simulink model "astatismo"  (R2026a)
settings: Solver=VariableStepAuto  StopTime=12  MaxStep=1e-2  RelTol=1e-6
undefined symbols (not defined in the file): A, B, C, C_theta, C_x, K_aum_2
settings Model: Creator=matte  LastModifiedBy=matte
settings OptimizationCC: BooleanDataType=off
settings DebuggingCC: SaveWithParameterizedLinksMsg=none  SignalResolutionControl=TryResolveAllWithWarning
settings HardwareCC: TargetUnknown=on

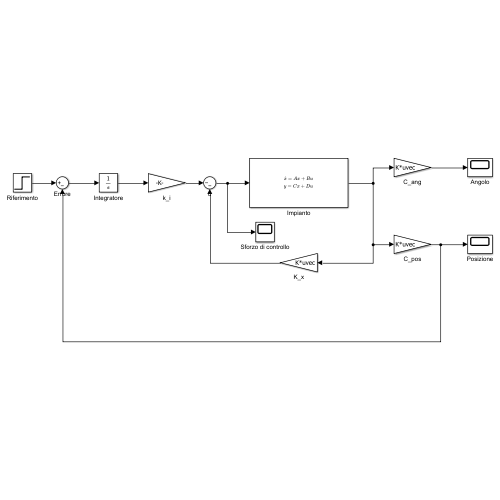
[thumbnail: Simulink's stored preview of the top-level diagram]
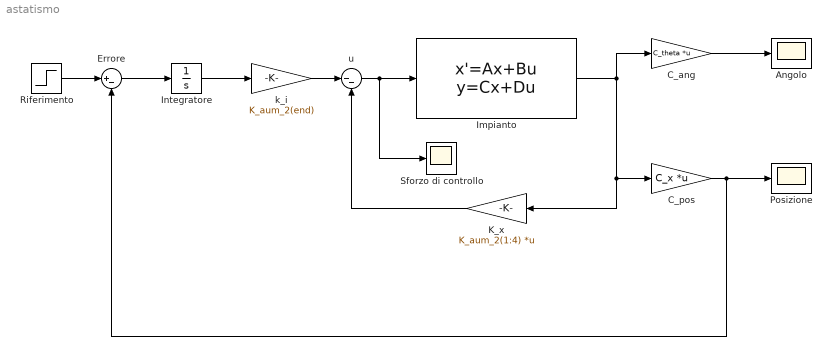
== system astatismo ==
  Angolo : Scope
      settings: ActiveDisplayYMinimum=-0.030053616149137433  ActiveDisplayYMaximum=0.040080838231526084
  C_ang : Gain  Gain=C_theta  Multiplication=Matrix(K*u) (u vector)
  C_pos : Gain  Gain=C_x  Multiplication=Matrix(K*u) (u vector)
  Errore : Sum  Inputs=|+-
  Impianto : StateSpace  A=A  B=B  C=C  D=zeros(4, 1)  InitialCondition=0
  Integratore : Integrator
  K_x : Gain  Gain=K_aum_2(1:4)  Multiplication=Matrix(K*u) (u vector)
  Posizione : Scope
      settings: ActiveDisplayYMinimum=-1  ActiveDisplayYMaximum=1
  Riferimento : Step  Time=0
  Sforzo di controllo : Scope
      settings: ActiveDisplayYMinimum=-0.059322755317915837  ActiveDisplayYMaximum=0.17371927600368323
  k_i : Gain  Gain=K_aum_2(end)
  u : Sum  Inputs=|--
  wires:
  Riferimento/1 -> Errore/1
  Errore/1 -> Integratore/1
  Integratore/1 -> k_i/1
  k_i/1 -> u/1
  u/1 -> Sforzo di controllo/1, Impianto/1
  Impianto/1 -> K_x/1, C_pos/1, C_ang/1
  K_x/1 -> u/2
  C_ang/1 -> Angolo/1
  C_pos/1 -> Posizione/1, Errore/2
